simulink model "CoETS_TrqCalc"  (R2016b)
settings: configuration reference "CodeGenConfigSet" (kept outside this file)
values from neighbouring files (symbols this model uses):
  CoETS_trqMaxOfsBrkDes_C = Calibration.Parameter    [init_CoETS_TrqCalc.m]    (also in init_CoETS_TrqCalc_SIL.m = Simulink.Parameter)
  CoETS_trqMinOfsBrkDes_C = Calibration.Parameter    [init_CoETS_TrqCalc.m]    (also in init_CoETS_TrqCalc_SIL.m = Simulink.Parameter)
  DCSOVRDSENGPRT_SY = fi(0,State_int32)    [init_CoETS_TrqCalc.m]    (also in init_CoETS_TrqCalc_SIL.m)
  ENGPRT_OVRDS_DCS = fi(1,State_int32)    [init_CoETS_TrqCalc.m]    (also in init_CoETS_TrqCalc_SIL.m)
  PTPRTOVRDSSPDGOV_SY = fi(0,State_int32)    [init_CoETS_TrqCalc.m]    (also in init_CoETS_TrqCalc_SIL.m)
  SPDGOV_OVRDS_PTPRT = fi(0,State_int32)    [init_CoETS_TrqCalc.m]    (also in init_CoETS_TrqCalc_SIL.m)
libraries: simulink x7
settings Model: Creator=Wollf  LastModifiedBy=xuxingpei
settings ConfigSetRef: SourceLocation=Base Workspace

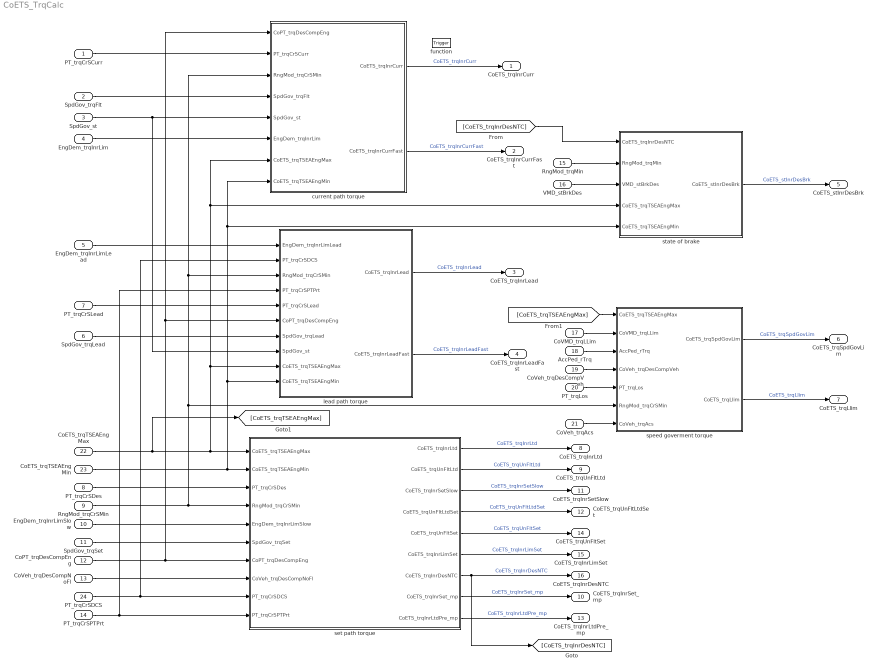
== system CoETS_TrqCalc ==
  PT_trqCrSCurr : Inport  Tag=Nm  Description=application parameter for lead torque order to engine for rail pressure control（crankshaft torque）  OutMin=-3000  OutMax=3000  OutDataTypeStr=Trq_Nm
  SpdGov_trqFlt : Inport  Tag=Nm  Description=filtered setpoint torque of SpdGov  Port=2  OutMin=-3267  OutMax=3267  OutDataTypeStr=Trq_Nm
  SpdGov_st : Inport  Description=status speed control SpdGov  Port=3  OutMin=0  OutMax=65535  OutDataTypeStr=State_uint16
  EngDem_trqInrLim : Inport  Tag=Nm  Description=Resulting limiting torque (inner engine torque)  Port=4  OutMin=-3276.8  OutMax=3276.7  OutDataTypeStr=Trq_Nm
  EngDem_trqInrLimLead : Inport  Tag=Nm  Description=inner engine limted lead torque  Port=5  OutMin=-3276.8  OutMax=3276.7  OutDataTypeStr=Trq_Nm
  SpdGov_trqLead : Inport  Tag=Nm  Description=lead torque of SpdGov on the air path  Port=6  OutMin=-3267  OutMax=3267  OutDataTypeStr=Trq_Nm
  PT_trqCrSLead : Inport  Tag=Nm  Description=application parameter for lead torque order to engine（crankshaft torque）  Port=7  OutMin=-3000  OutMax=3000  OutDataTypeStr=Trq_Nm
  PT_trqCrSDes : Inport  Tag=Nm  Description=Application parameter for requested propulsion torque to engine(crankshaft torque)  Port=8  OutMin=-3000  OutMax=3000  OutDataTypeStr=Trq_Nm
  RngMod_trqCrSMin : Inport  Tag=Nm  Description=minimal crankshaft torque  Port=9  OutMin=-3276.8  OutMax=3276.7  OutDataTypeStr=Trq_Nm
  EngDem_trqInrLimSlow : Inport  Tag=Nm  Description=inner engine limted torque for Slow Path  Port=10  OutMin=-3276.8  OutMax=3276.7  OutDataTypeStr=Trq_Nm
  SpdGov_trqSet : Inport  Tag=Nm  Description=Set point torque of SpdGov on the fuel path  Port=11  OutMin=-3000  OutMax=3000  OutDataTypeStr=Trq_Nm
  CoPT_trqDesCompEng : Inport  Tag=Nm  Description=Application parameter for engine torque desired for compensation  Port=12  OutMin=-3276  OutMax=3276  OutDataTypeStr=Trq_Nm
  CoVeh_trqDesCompNoFl : Inport  Tag=Nm  Description=compensation torque with the shares,which not slur by the drive behaviour filter  Port=13  OutMin=-3000  OutMax=3000  OutDataTypeStr=Trq_Nm
  PT_trqCrSPTPrt : Inport  Tag=Nm  Description=Application parameter for powertrain protection train protection torque(crankshaft torque)  Port=14  OutMin=-3000  OutMax=3000  OutDataTypeStr=Trq_Nm
  RngMod_trqMin : Inport  Tag=Nm  Description=Drag torque (minimum torque)  Port=15  OutMin=-3276.8  OutMax=3276.7  OutDataTypeStr=Trq_Nm
  VMD_stBrkDes : Inport  Description=Application parameter for torque status information  Port=16  OutMin=0  OutMax=65535  OutDataTypeStr=State_uint16
  CoVMD_trqLLim : Inport  Tag=Nm  Description=propulsion torque of longitudinal limter  Port=17  OutMin=-3000  OutMax=3000  OutDataTypeStr=Trq_Nm
  AccPed_rTrq : Inport  Description=Total drive train ratio of engine - wheel  Port=18  OutMin=-327  OutMax=327  OutDataTypeStr=TransRatio
  CoVeh_trqDesCompVeh : Inport  Tag=Nm  Description=Signal for compensation correction of wheel torque level (signal 1)  Port=19  OutMin=-3000  OutMax=3000  OutDataTypeStr=Trq_Nm
  PT_trqLos : Inport  Tag=Nm  Description=Parameter for loss torque of the drive train  Port=20  OutMin=-3000  OutMax=3000  OutDataTypeStr=Trq_Nm
  CoVeh_trqAcs : Inport  Tag=Nm  Description=message for demand of accessories  Port=21  OutMin=-3276.8  OutMax=3276.7  OutDataTypeStr=Trq_Nm
  CoETS_trqTSEAEngMax : Inport  Tag=Nm  Description=torque request to engine intervention decrement(Max)  Port=22  OutMin=-3276  OutMax=3276  OutDataTypeStr=Trq_Nm
  CoETS_trqTSEAEngMin : Inport  Tag=Nm  Description=torque request to engine intervention increment(Min)  Port=23  OutMin=-3276  OutMax=3276  OutDataTypeStr=Trq_Nm
  PT_trqCrSDCS : Inport  Tag=Nm  Description=crankshaft torque for request decrcment  Port=24  OutMin=-3000  OutMax=3000  OutDataTypeStr=Trq_Nm
  function : TriggerPort  TriggerType=function-call  VariantControl=Variant
  current path torque : Subsystem
  lead path torque : Subsystem
  set path torque : Subsystem
  speed goverment torque : Subsystem
  state of brake : Subsystem
  CoETS_trqInrCurr : Outport  Tag=Nm  Description=Inner torque current value  OutMin=-3276  OutMax=3276  OutDataTypeStr=Trq_Nm
  CoETS_trqInrCurrFast : Outport  Tag=Nm  Description=Inner desired torque (fast path) calculated from CoPT_trqCurrEng [Nm]  Port=2  OutMin=-3276  OutMax=3276  OutDataTypeStr=Trq_Nm
  CoETS_trqInrLead : Outport  Tag=Nm  Description=desired lead (inner) torque (without Filter with reserve)  Port=3  OutMin=-3276  OutMax=3276  OutDataTypeStr=Trq_Nm
  CoETS_trqInrLeadFast : Outport  Tag=Nm  Description=Inner torque desired value (fast signal path) generated out of CoPT_trqLeadEng  Port=4  OutMin=-3276  OutMax=3276  OutDataTypeStr=Trq_Nm
  CoETS_stInrDesBrk : Outport  Description=Negative torque status for inner torque  Port=5  OutMin=0  OutMax=4294967295  OutDataTypeStr=State_uint32
  CoETS_trqSpdGovLim : Outport  Tag=Nm  Description=Inner engine limitation torque for EISGov  Port=6  OutMin=-3276.8  OutMax=3276.7  OutDataTypeStr=Trq_Nm
  CoETS_trqLlim : Outport  Tag=Nm  Description=Longitudinal limitation for inner engine torque  Port=7  OutMin=-3276  OutMax=3276  OutDataTypeStr=Trq_Nm
  CoETS_trqInrLtd : Outport  Tag=Nm  Description=inner torque set value after limitation, before AS  Port=8  OutMin=-3000  OutMax=3000  OutDataTypeStr=Trq_Nm
  CoETS_trqUnFltLtd : Outport  Tag=Nm  Description=Limited idle speed governor torque  Port=9  OutMin=-3276  OutMax=3276  OutDataTypeStr=Trq_Nm
  CoETS_trqInrSet_mp : Outport  Tag=Nm  Description=Intermediate inner torque for the set path without filteration  Port=10  OutMin=-3276  OutMax=3276  OutDataTypeStr=Trq_Nm
  CoETS_trqInrSetSlow : Outport  Tag=Nm  Description=Filtered inner torque ( positive torque) desired value (standard signal path) generated out of CoPT_trqDesEng  Port=11  OutMin=-3276  OutMax=3276  OutDataTypeStr=Trq_Nm
  CoETS_trqUnFltLtdSet : Outport  Tag=Nm  Description=Compensation torque of the accessories  Port=12  OutMin=-3276  OutMax=3276  OutDataTypeStr=Trq_Nm
  CoETS_trqInrLtdPre_mp : Outport  Tag=Nm  Description=inner set torque after limitation, before active surge damper  Port=13  OutMin=-3276  OutMax=3276  OutDataTypeStr=Trq_Nm
  CoETS_trqUnFltSet : Outport  Tag=Nm  Description="Compensation torque of \"loss torque compensation\" to bypass filter influences on the set path which is partly compensated"  Port=14  OutMin=-3276  OutMax=3276  OutDataTypeStr=Trq_Nm
  CoETS_trqInrLimSet : Outport  Tag=Nm  Description=Limitation torque without the part of the speed governor  Port=15  OutMin=-3000  OutMax=3000  OutDataTypeStr=Trq_Nm
  CoETS_trqInrDesNTC : Outport  Tag=Nm  Description=Additional desired engine friction Nm  Port=16  OutMin=-3276  OutMax=3276  OutDataTypeStr=Trq_Nm
  wires:
  RngMod_trqMin/1 -> state of brake/2(RngMod_trqMin)
  SpdGov_st/1 -> lead path torque/8(SpdGov_st), current path torque/5(SpdGov_st)
  SpdGov_trqFlt/1 -> current path torque/4(SpdGov_trqFlt)
  EngDem_trqInrLim/1 -> current path torque/6(EngDem_trqInrLim)
  VMD_stBrkDes/1 -> state of brake/3(VMD_stBrkDes)
  state of brake/1(CoETS_stInrDesBrk) -> CoETS_stInrDesBrk/1  "CoETS_stInrDesBrk"
  current path torque/1(CoETS_trqInrCurr) -> CoETS_trqInrCurr/1  "CoETS_trqInrCurr"
  AccPed_rTrq/1 -> speed goverment torque/3(AccPed_rTrq)
  CoVeh_trqAcs/1 -> speed goverment torque/7(CoVeh_trqAcs)
  CoVMD_trqLLim/1 -> speed goverment torque/2(CoVMD_trqLLim)
  speed goverment torque/1(CoETS_trqSpdGovLim) -> CoETS_trqSpdGovLim/1  "CoETS_trqSpdGovLim"
  CoVeh_trqDesCompVeh/1 -> speed goverment torque/4(CoVeh_trqDesCompVeh)
  PT_trqLos/1 -> speed goverment torque/5(PT_trqLos)
  lead path torque/1(CoETS_trqInrLead) -> CoETS_trqInrLead/1  "CoETS_trqInrLead"
  PT_trqCrSCurr/1 -> current path torque/2(PT_trqCrSCurr)
  EngDem_trqInrLimLead/1 -> lead path torque/1(EngDem_trqInrLimLead)
  RngMod_trqCrSMin/1 -> current path torque/3(RngMod_trqCrSMin), lead path torque/3(RngMod_trqCrSMin), speed goverment torque/6(RngMod_trqCrSMin), set path torque/4(RngMod_trqCrSMin)
  CoPT_trqDesCompEng/1 -> current path torque/1(CoPT_trqDesCompEng), lead path torque/6(CoPT_trqDesCompEng), set path torque/7(CoPT_trqDesCompEng)
  PT_trqCrSPTPrt/1 -> lead path torque/4(PT_trqCrSPTPrt), set path torque/10(PT_trqCrSPTPrt)
  CoETS_trqTSEAEngMin/1 -> current path torque/8(CoETS_trqTSEAEngMin), state of brake/5(CoETS_trqTSEAEngMin), lead path torque/10(CoETS_trqTSEAEngMin), set path torque/2(CoETS_trqTSEAEngMin)
  CoETS_trqTSEAEngMax/1 -> [CoETS_trqTSEAEngMax], current path torque/7(CoETS_trqTSEAEngMax), state of brake/4(CoETS_trqTSEAEngMax), lead path torque/9(CoETS_trqTSEAEngMax), set path torque/1(CoETS_trqTSEAEngMax)
  [CoETS_trqInrDesNTC] -> state of brake/1(CoETS_trqInrDesNTC)
  current path torque/2(CoETS_trqInrCurrFast) -> CoETS_trqInrCurrFast/1  "CoETS_trqInrCurrFast"
  lead path torque/2(CoETS_trqInrLeadFast) -> CoETS_trqInrLeadFast/1  "CoETS_trqInrLeadFast"
  speed goverment torque/2(CoETS_trqLlim) -> CoETS_trqLlim/1  "CoETS_trqLlim"
  PT_trqCrSDes/1 -> set path torque/3(PT_trqCrSDes)
  EngDem_trqInrLimSlow/1 -> set path torque/5(EngDem_trqInrLimSlow)
  SpdGov_trqSet/1 -> set path torque/6(SpdGov_trqSet)
  CoVeh_trqDesCompNoFl/1 -> set path torque/8(CoVeh_trqDesCompNoFl)
  set path torque/2(CoETS_trqUnFltLtd) -> CoETS_trqUnFltLtd/1  "CoETS_trqUnFltLtd"
  set path torque/9(CoETS_trqInrLtdPre_mp) -> CoETS_trqInrLtdPre_mp/1  "CoETS_trqInrLtdPre_mp"
  set path torque/6(CoETS_trqInrLimSet) -> CoETS_trqInrLimSet/1  "CoETS_trqInrLimSet"
  set path torque/7(CoETS_trqInrDesNTC) -> CoETS_trqInrDesNTC/1, [CoETS_trqInrDesNTC]  "CoETS_trqInrDesNTC"
  [CoETS_trqTSEAEngMax] -> speed goverment torque/1(CoETS_trqTSEAEngMax)
  set path torque/8(CoETS_trqInrSet_mp) -> CoETS_trqInrSet_mp/1  "CoETS_trqInrSet_mp"
  set path torque/3(CoETS_trqInrSetSlow) -> CoETS_trqInrSetSlow/1  "CoETS_trqInrSetSlow"
  set path torque/1(CoETS_trqInrLtd) -> CoETS_trqInrLtd/1  "CoETS_trqInrLtd"
  PT_trqCrSDCS/1 -> lead path torque/2(PT_trqCrSDCS), set path torque/9(PT_trqCrSDCS)
  set path torque/4(CoETS_trqUnFltLtdSet) -> CoETS_trqUnFltLtdSet/1  "CoETS_trqUnFltLtdSet"
  set path torque/5(CoETS_trqUnFltSet) -> CoETS_trqUnFltSet/1  "CoETS_trqUnFltSet"
  SpdGov_trqLead/1 -> lead path torque/7(SpdGov_trqLead)
  PT_trqCrSLead/1 -> lead path torque/5(PT_trqCrSLead)

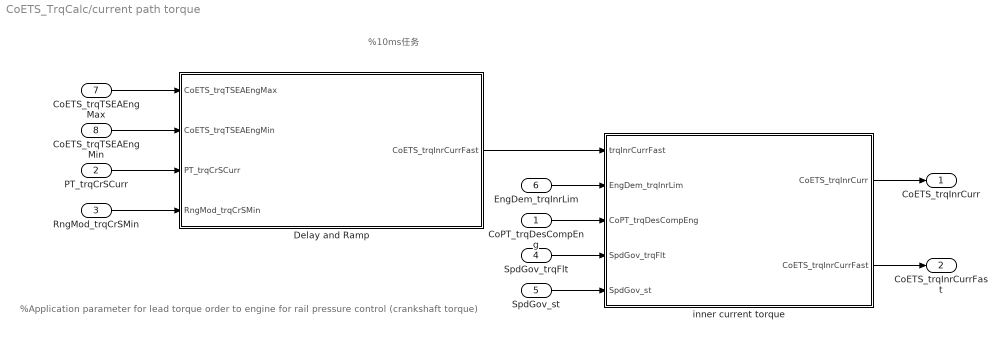
== system CoETS_TrqCalc/current path torque ==
  note: %10ms任务
  note: %Application parameter for lead torque order to engine for rail pressure control (crankshaft torque)
  CoPT_trqDesCompEng : Inport
  PT_trqCrSCurr : Inport  Port=2
  RngMod_trqCrSMin : Inport  Port=3
  SpdGov_trqFlt : Inport  Port=4
  SpdGov_st : Inport  Port=5
  EngDem_trqInrLim : Inport  Port=6
  CoETS_trqTSEAEngMax : Inport  Port=7
  CoETS_trqTSEAEngMin : Inport  Port=8
  Delay and Ramp : Subsystem
  inner current torque : Subsystem
  CoETS_trqInrCurr : Outport
  CoETS_trqInrCurrFast : Outport  Port=2
  wires:
  RngMod_trqCrSMin/1 -> Delay and Ramp/4(RngMod_trqCrSMin)
  PT_trqCrSCurr/1 -> Delay and Ramp/3(PT_trqCrSCurr)
  CoETS_trqTSEAEngMin/1 -> Delay and Ramp/2(CoETS_trqTSEAEngMin)
  CoETS_trqTSEAEngMax/1 -> Delay and Ramp/1(CoETS_trqTSEAEngMax)
  Delay and Ramp/1(CoETS_trqInrCurrFast) -> inner current torque/1(trqInrCurrFast)
  EngDem_trqInrLim/1 -> inner current torque/2(EngDem_trqInrLim)
  CoPT_trqDesCompEng/1 -> inner current torque/3(CoPT_trqDesCompEng)
  SpdGov_trqFlt/1 -> inner current torque/4(SpdGov_trqFlt)
  SpdGov_st/1 -> inner current torque/5(SpdGov_st)
  inner current torque/1(CoETS_trqInrCurr) -> CoETS_trqInrCurr/1
  inner current torque/2(CoETS_trqInrCurrFast) -> CoETS_trqInrCurrFast/1

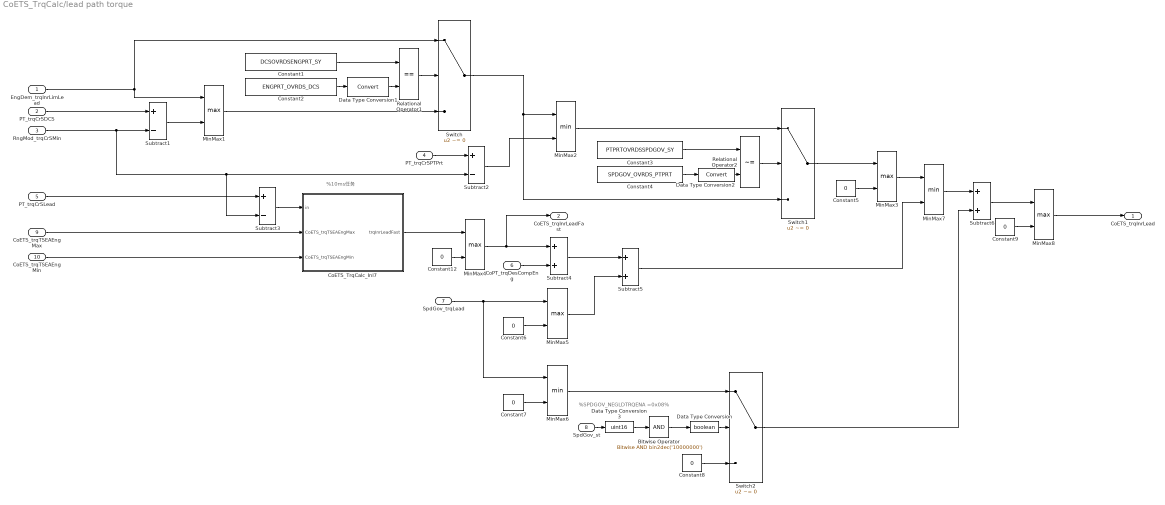
== system CoETS_TrqCalc/lead path torque ==
  note: %10ms任务
  note: %SPDGOV_NEGLDTRQENA =0x08%
  EngDem_trqInrLimLead : Inport
  PT_trqCrSDCS : Inport  Port=2
  RngMod_trqCrSMin : Inport  Port=3
  PT_trqCrSPTPrt : Inport  Port=4
  PT_trqCrSLead : Inport  Port=5
  CoPT_trqDesCompEng : Inport  Port=6
  SpdGov_trqLead : Inport  Port=7
  SpdGov_st : Inport  Port=8
  CoETS_trqTSEAEngMax : Inport  Port=9
  CoETS_trqTSEAEngMin : Inport  Port=10
  Bitwise Operator : simulink/Logic and Bit Operations/Bitwise Operator  logicop=AND  UseBitMask=on  BitMask=bin2dec('10000000')  BitMaskRealWorld=Stored Integer
  CoETS_TrqCalc_Inl7 : Subsystem
  Constant1 : Constant  Value=DCSOVRDSENGPRT_SY  VectorParams1D=off
  Constant{5..9,12} (6 alike) : Constant  Value=0  VectorParams1D=off  OutDataTypeStr=Inherit: Inherit via back propagation
  Constant2 : Constant  Value=ENGPRT_OVRDS_DCS  VectorParams1D=off
  Constant3 : Constant  Value=PTPRTOVRDSSPDGOV_SY  VectorParams1D=off
  Constant4 : Constant  Value=SPDGOV_OVRDS_PTPRT  VectorParams1D=off
  Data Type Conversion : DataTypeConversion  OutDataTypeStr=boolean
  Data Type Conversion1 : DataTypeConversion
  Data Type Conversion2 : DataTypeConversion
  Data Type Conversion3 : DataTypeConversion  OutDataTypeStr=uint16
  MinMax{1,3..5,8} (5 alike) : MinMax  Function=max  Inputs=2  InputSameDT=on
  MinMax2 : MinMax  Inputs=2  InputSameDT=on
  MinMax6 : MinMax  Inputs=2  InputSameDT=on
  MinMax7 : MinMax  Inputs=2  InputSameDT=on
  Relational Operator1 : RelationalOperator  Operator===  OutDataTypeStr=boolean  RndMeth=Simplest  InputSameDT=on
  Relational Operator2 : RelationalOperator  Operator=~=  OutDataTypeStr=boolean  RndMeth=Simplest  InputSameDT=on
  Subtract1 : Sum  Inputs=+-  OutDataTypeStr=Inherit: Inherit via back propagation  SaturateOnIntegerOverflow=on  InputSameDT=on
  Subtract2 : Sum  Inputs=+-  OutDataTypeStr=Inherit: Inherit via back propagation  SaturateOnIntegerOverflow=on  InputSameDT=on
  Subtract3 : Sum  Inputs=+-  OutDataTypeStr=Inherit: Inherit via back propagation  SaturateOnIntegerOverflow=on  InputSameDT=on
  Subtract4 : Sum  OutDataTypeStr=Inherit: Inherit via back propagation  SaturateOnIntegerOverflow=on  InputSameDT=on
  Subtract5 : Sum  OutDataTypeStr=Inherit: Inherit via back propagation  SaturateOnIntegerOverflow=on  InputSameDT=on
  Subtract6 : Sum  OutDataTypeStr=Inherit: Inherit via back propagation  SaturateOnIntegerOverflow=on  InputSameDT=on
  Switch : Switch  Criteria=u2 ~= 0  OutDataTypeStr=Inherit: Inherit via back propagation  SaturateOnIntegerOverflow=on  InputSameDT=on
  Switch1 : Switch  Criteria=u2 ~= 0  OutDataTypeStr=Inherit: Inherit via back propagation  SaturateOnIntegerOverflow=on  InputSameDT=on
  Switch2 : Switch  Criteria=u2 ~= 0  OutDataTypeStr=Inherit: Inherit via back propagation  SaturateOnIntegerOverflow=on  InputSameDT=on
  CoETS_trqInrLead : Outport
  CoETS_trqInrLeadFast : Outport  Port=2
  wires:
  EngDem_trqInrLimLead/1 -> MinMax1/1, Switch/1
  Subtract1/1 -> MinMax1/2
  MinMax1/1 -> Switch/3
  Data Type Conversion2/1 -> Relational Operator2/2
  Data Type Conversion1/1 -> Relational Operator1/2
  CoETS_trqTSEAEngMin/1 -> CoETS_TrqCalc_Inl7/3(CoETS_trqTSEAEngMin)
  CoETS_trqTSEAEngMax/1 -> CoETS_TrqCalc_Inl7/2(CoETS_trqTSEAEngMax)
  MinMax8/1 -> CoETS_trqInrLead/1
  Constant9/1 -> MinMax8/2
  Subtract6/1 -> MinMax8/1
  Switch2/1 -> Subtract6/2
  MinMax7/1 -> Subtract6/1
  Subtract5/1 -> MinMax7/2
  MinMax3/1 -> MinMax7/1
  Constant8/1 -> Switch2/3
  Data Type Conversion/1 -> Switch2/2
  Bitwise Operator/1 -> Data Type Conversion/1
  SpdGov_st/1 -> Data Type Conversion3/1
  MinMax6/1 -> Switch2/1
  MinMax5/1 -> Subtract5/2
  Subtract4/1 -> Subtract5/1
  SpdGov_trqLead/1 -> MinMax5/1, MinMax6/1
  Constant7/1 -> MinMax6/2
  Constant6/1 -> MinMax5/2
  CoPT_trqDesCompEng/1 -> Subtract4/2
  MinMax4/1 -> Subtract4/1, CoETS_trqInrLeadFast/1
  Constant12/1 -> MinMax4/2
  CoETS_TrqCalc_Inl7/1(trqInrLeadFast) -> MinMax4/1
  Subtract3/1 -> CoETS_TrqCalc_Inl7/1(in)
  PT_trqCrSLead/1 -> Subtract3/1
  Constant5/1 -> MinMax3/2
  Switch1/1 -> MinMax3/1
  MinMax2/1 -> Switch1/1
  Subtract2/1 -> MinMax2/2
  PT_trqCrSPTPrt/1 -> Subtract2/1
  Switch/1 -> MinMax2/1, Switch1/3
  RngMod_trqCrSMin/1 -> Subtract1/2, Subtract3/2, Subtract2/2
  PT_trqCrSDCS/1 -> Subtract1/1
  Relational Operator2/1 -> Switch1/2
  Relational Operator1/1 -> Switch/2
  Constant4/1 -> Data Type Conversion2/1
  Constant3/1 -> Relational Operator2/1
  Constant2/1 -> Data Type Conversion1/1
  Constant1/1 -> Relational Operator1/1
  Data Type Conversion3/1 -> Bitwise Operator/1

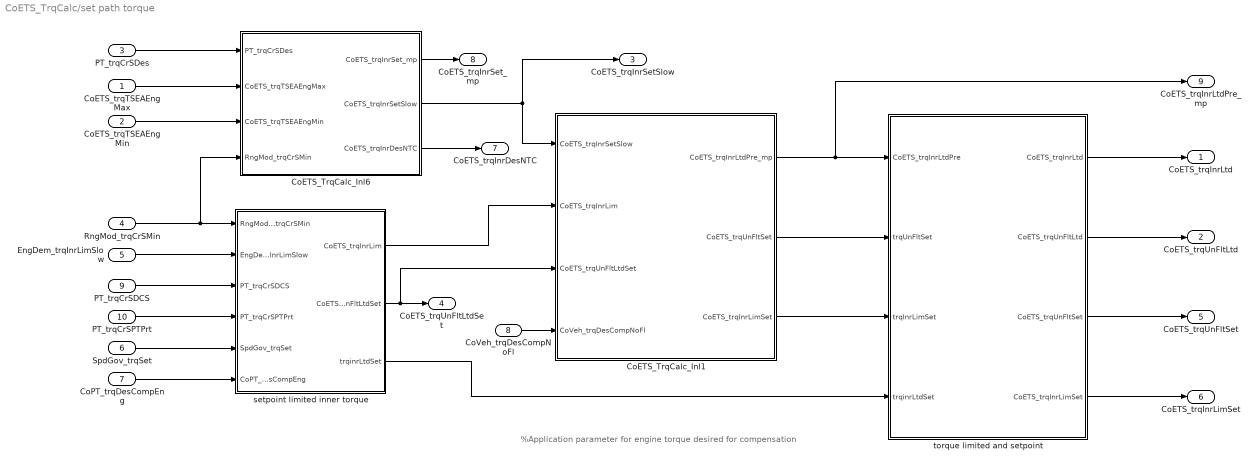
== system CoETS_TrqCalc/set path torque ==
  note: %Application parameter for engine torque desired for compensation
  CoETS_trqTSEAEngMax : Inport
  CoETS_trqTSEAEngMin : Inport  Port=2
  PT_trqCrSDes : Inport  Port=3
  RngMod_trqCrSMin : Inport  Port=4
  EngDem_trqInrLimSlow : Inport  Port=5
  SpdGov_trqSet : Inport  Port=6
  CoPT_trqDesCompEng : Inport  Port=7
  CoVeh_trqDesCompNoFl : Inport  Port=8
  PT_trqCrSDCS : Inport  Port=9
  PT_trqCrSPTPrt : Inport  Port=10
  CoETS_TrqCalc_Inl1 : Subsystem
  CoETS_TrqCalc_Inl6 : Subsystem
  setpoint limited inner torque : Subsystem
  torque limited and setpoint : Subsystem
  CoETS_trqInrLtd : Outport
  CoETS_trqUnFltLtd : Outport  Port=2
  CoETS_trqInrSetSlow : Outport  Port=3
  CoETS_trqUnFltLtdSet : Outport  Port=4
  CoETS_trqUnFltSet : Outport  Port=5
  CoETS_trqInrLimSet : Outport  Port=6
  CoETS_trqInrDesNTC : Outport  Port=7
  CoETS_trqInrSet_mp : Outport  Port=8
  CoETS_trqInrLtdPre_mp : Outport  Port=9
  wires:
  RngMod_trqCrSMin/1 -> CoETS_TrqCalc_Inl6/4(RngMod_trqCrSMin), setpoint limited inner torque/1(RngMod_trqCrSMin)
  PT_trqCrSDes/1 -> CoETS_TrqCalc_Inl6/1(PT_trqCrSDes)
  CoETS_trqTSEAEngMax/1 -> CoETS_TrqCalc_Inl6/2(CoETS_trqTSEAEngMax)
  CoETS_trqTSEAEngMin/1 -> CoETS_TrqCalc_Inl6/3(CoETS_trqTSEAEngMin)
  CoVeh_trqDesCompNoFl/1 -> CoETS_TrqCalc_Inl1/4(CoVeh_trqDesCompNoFl)
  setpoint limited inner torque/2(CoETS_trqUnFltLtdSet) -> CoETS_trqUnFltLtdSet/1, CoETS_TrqCalc_Inl1/3(CoETS_trqUnFltLtdSet)
  EngDem_trqInrLimSlow/1 -> setpoint limited inner torque/2(EngDem_trqInrLimSlow)
  PT_trqCrSDCS/1 -> setpoint limited inner torque/3(PT_trqCrSDCS)
  PT_trqCrSPTPrt/1 -> setpoint limited inner torque/4(PT_trqCrSPTPrt)
  SpdGov_trqSet/1 -> setpoint limited inner torque/5(SpdGov_trqSet)
  CoPT_trqDesCompEng/1 -> setpoint limited inner torque/6(CoPT_trqDesCompEng)
  setpoint limited inner torque/1(CoETS_trqInrLim) -> CoETS_TrqCalc_Inl1/2(CoETS_trqInrLim)
  CoETS_TrqCalc_Inl6/1(CoETS_trqInrSet_mp) -> CoETS_trqInrSet_mp/1
  CoETS_TrqCalc_Inl6/2(CoETS_trqInrSetSlow) -> CoETS_trqInrSetSlow/1, CoETS_TrqCalc_Inl1/1(CoETS_trqInrSetSlow)
  CoETS_TrqCalc_Inl6/3(CoETS_trqInrDesNTC) -> CoETS_trqInrDesNTC/1
  CoETS_TrqCalc_Inl1/1(CoETS_trqInrLtdPre_mp) -> CoETS_trqInrLtdPre_mp/1, torque limited and setpoint/1(CoETS_trqInrLtdPre)
  CoETS_TrqCalc_Inl1/2(CoETS_trqUnFltSet) -> torque limited and setpoint/2(trqUnFltSet)
  CoETS_TrqCalc_Inl1/3(CoETS_trqInrLimSet) -> torque limited and setpoint/3(trqInrLimSet)
  setpoint limited inner torque/3(trqinrLtdSet) -> torque limited and setpoint/4(trqinrLtdSet)
  torque limited and setpoint/1(CoETS_trqInrLtd) -> CoETS_trqInrLtd/1
  torque limited and setpoint/2(CoETS_trqUnFltLtd) -> CoETS_trqUnFltLtd/1
  torque limited and setpoint/3(CoETS_trqUnFltSet) -> CoETS_trqUnFltSet/1
  torque limited and setpoint/4(CoETS_trqInrLimSet) -> CoETS_trqInrLimSet/1

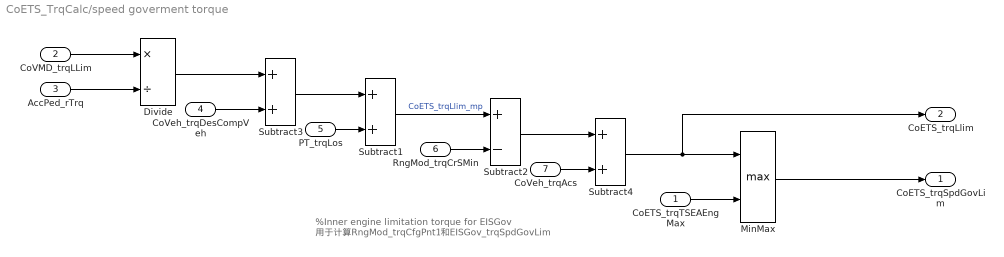
== system CoETS_TrqCalc/speed goverment torque ==
  note: %Inner engine limitation torque for EISGov
      | 用于计算RngMod_trqCfgPnt1和EISGov_trqSpdGovLim
  CoETS_trqTSEAEngMax : Inport
  CoVMD_trqLLim : Inport  Port=2
  AccPed_rTrq : Inport  Port=3
  CoVeh_trqDesCompVeh : Inport  Port=4
  PT_trqLos : Inport  Port=5
  RngMod_trqCrSMin : Inport  Port=6
  CoVeh_trqAcs : Inport  Port=7
  Divide : Product  Inputs=*/  OutDataTypeStr=Inherit: Inherit via back propagation  SaturateOnIntegerOverflow=on
  MinMax : MinMax  Function=max  Inputs=2  InputSameDT=on
  Subtract1 : Sum  OutDataTypeStr=Inherit: Inherit via back propagation  SaturateOnIntegerOverflow=on  InputSameDT=on
  Subtract2 : Sum  Inputs=+-  OutDataTypeStr=Inherit: Inherit via back propagation  SaturateOnIntegerOverflow=on  InputSameDT=on
  Subtract3 : Sum  OutDataTypeStr=Inherit: Inherit via back propagation  SaturateOnIntegerOverflow=on  InputSameDT=on
  Subtract4 : Sum  OutDataTypeStr=Inherit: Inherit via back propagation  SaturateOnIntegerOverflow=on  InputSameDT=on
  CoETS_trqSpdGovLim : Outport
  CoETS_trqLlim : Outport  Port=2
  wires:
  MinMax/1 -> CoETS_trqSpdGovLim/1
  CoETS_trqTSEAEngMax/1 -> MinMax/2
  Subtract4/1 -> MinMax/1, CoETS_trqLlim/1
  CoVeh_trqAcs/1 -> Subtract4/2
  Subtract2/1 -> Subtract4/1
  RngMod_trqCrSMin/1 -> Subtract2/2
  Subtract1/1 -> Subtract2/1  "CoETS_trqLlim_mp"
  PT_trqLos/1 -> Subtract1/2
  Subtract3/1 -> Subtract1/1
  CoVeh_trqDesCompVeh/1 -> Subtract3/2
  Divide/1 -> Subtract3/1
  AccPed_rTrq/1 -> Divide/2
  CoVMD_trqLLim/1 -> Divide/1

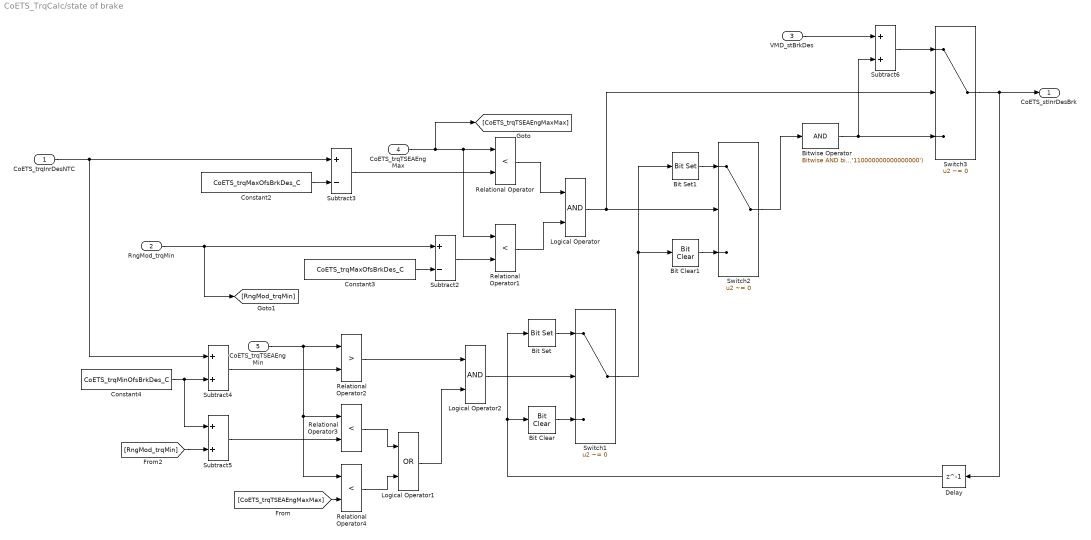
== system CoETS_TrqCalc/state of brake ==
  CoETS_trqInrDesNTC : Inport
  RngMod_trqMin : Inport  Port=2
  VMD_stBrkDes : Inport  Port=3
  CoETS_trqTSEAEngMax : Inport  Port=4
  CoETS_trqTSEAEngMin : Inport  Port=5
  Bit Clear : simulink/Logic and Bit Operations/Bit Clear  iBit=17
  Bit Clear1 : simulink/Logic and Bit Operations/Bit Clear  iBit=16
  Bit Set : simulink/Logic and Bit Operations/Bit Set  iBit=17
  Bit Set1 : simulink/Logic and Bit Operations/Bit Set  iBit=16
  Bitwise Operator : simulink/Logic and Bit Operations/Bitwise Operator  logicop=AND  UseBitMask=on  BitMask=bin2dec('110000000000000000')  BitMaskRealWorld=Stored Integer
  Constant2 : Constant  Value=CoETS_trqMaxOfsBrkDes_C  VectorParams1D=off
  Constant3 : Constant  Value=CoETS_trqMaxOfsBrkDes_C  VectorParams1D=off
  Constant4 : Constant  Value=CoETS_trqMinOfsBrkDes_C  VectorParams1D=off
  Delay : Delay  DelayLength=1  InitialCondition=0
  Logical Operator : Logic  AllPortsSameDT=off  OutDataTypeStr=boolean
  Logical Operator1 : Logic  Operator=OR  AllPortsSameDT=off  OutDataTypeStr=boolean
  Logical Operator2 : Logic  AllPortsSameDT=off  OutDataTypeStr=boolean
  Relational Operator{,1,3..4} (4 alike) : RelationalOperator  Operator=<  OutDataTypeStr=boolean  RndMeth=Simplest  InputSameDT=on
  Relational Operator2 : RelationalOperator  Operator=>  OutDataTypeStr=boolean  RndMeth=Simplest  InputSameDT=on
  Subtract2 : Sum  Inputs=+-  OutDataTypeStr=Inherit: Inherit via back propagation  SaturateOnIntegerOverflow=on  InputSameDT=on
  Subtract3 : Sum  Inputs=+-  OutDataTypeStr=Inherit: Inherit via back propagation  SaturateOnIntegerOverflow=on  InputSameDT=on
  Subtract4 : Sum  OutDataTypeStr=Inherit: Inherit via back propagation  SaturateOnIntegerOverflow=on  InputSameDT=on
  Subtract5 : Sum  OutDataTypeStr=Inherit: Inherit via back propagation  SaturateOnIntegerOverflow=on  InputSameDT=on
  Subtract6 : Sum  OutDataTypeStr=Inherit: Inherit via back propagation  SaturateOnIntegerOverflow=on
  Switch1 : Switch  Criteria=u2 ~= 0  OutDataTypeStr=Inherit: Inherit via back propagation  SaturateOnIntegerOverflow=on  InputSameDT=on
  Switch2 : Switch  Criteria=u2 ~= 0  OutDataTypeStr=Inherit: Inherit via back propagation  SaturateOnIntegerOverflow=on  InputSameDT=on
  Switch3 : Switch  Criteria=u2 ~= 0  OutDataTypeStr=Inherit: Inherit via back propagation  SaturateOnIntegerOverflow=on  InputSameDT=on
  CoETS_stInrDesBrk : Outport
  wires:
  Delay/1 -> Bit Clear/1, Bit Set/1
  VMD_stBrkDes/1 -> Subtract6/1
  Switch2/1 -> Bitwise Operator/1
  Bitwise Operator/1 -> Switch3/3, Subtract6/2
  Subtract6/1 -> Switch3/1
  Switch1/1 -> Bit Clear1/1, Bit Set1/1
  Bit Clear1/1 -> Switch2/3
  Bit Set1/1 -> Switch2/1
  Logical Operator/1 -> Switch2/2, Switch3/2
  Bit Clear/1 -> Switch1/3
  Switch3/1 -> CoETS_stInrDesBrk/1, Delay/1
  Bit Set/1 -> Switch1/1
  Logical Operator2/1 -> Switch1/2
  Logical Operator1/1 -> Logical Operator2/2
  Relational Operator2/1 -> Logical Operator2/1
  Relational Operator3/1 -> Logical Operator1/1
  Relational Operator4/1 -> Logical Operator1/2
  Subtract5/1 -> Relational Operator3/2
  CoETS_trqTSEAEngMin/1 -> Relational Operator2/1, Relational Operator3/1, Relational Operator4/1
  Subtract4/1 -> Relational Operator2/2
  Constant4/1 -> Subtract4/2, Subtract5/1
  CoETS_trqInrDesNTC/1 -> Subtract4/1, Subtract3/1
  Relational Operator1/1 -> Logical Operator/2
  Subtract2/1 -> Relational Operator1/2
  Constant3/1 -> Subtract2/2
  RngMod_trqMin/1 -> [RngMod_trqMin], Subtract2/1
  Relational Operator/1 -> Logical Operator/1
  CoETS_trqTSEAEngMax/1 -> [CoETS_trqTSEAEngMaxMax], Relational Operator/1, Relational Operator1/1
  Subtract3/1 -> Relational Operator/2
  Constant2/1 -> Subtract3/2
  [CoETS_trqTSEAEngMaxMax] -> Relational Operator4/2
  [RngMod_trqMin] -> Subtract5/2

== system CoETS_TrqCalc/current path torque/Delay and Ramp ==
  CoETS_trqTSEAEngMax : Inport
  CoETS_trqTSEAEngMin : Inport  Port=2
  PT_trqCrSCurr : Inport  Port=3
  RngMod_trqCrSMin : Inport  Port=4
  MinMax2 : MinMax  Inputs=2  InputSameDT=on
  MinMax3 : MinMax  Function=max  Inputs=2  InputSameDT=on
  Subtract3 : Sum  Inputs=+-  OutDataTypeStr=Inherit: Inherit via back propagation  SaturateOnIntegerOverflow=on  InputSameDT=on
  CoETS_trqInrCurrFast : Outport
  wires:
  MinMax3/1 -> CoETS_trqInrCurrFast/1
  CoETS_trqTSEAEngMin/1 -> MinMax3/2
  MinMax2/1 -> MinMax3/1
  CoETS_trqTSEAEngMax/1 -> MinMax2/1
  Subtract3/1 -> MinMax2/2
  RngMod_trqCrSMin/1 -> Subtract3/2
  PT_trqCrSCurr/1 -> Subtract3/1

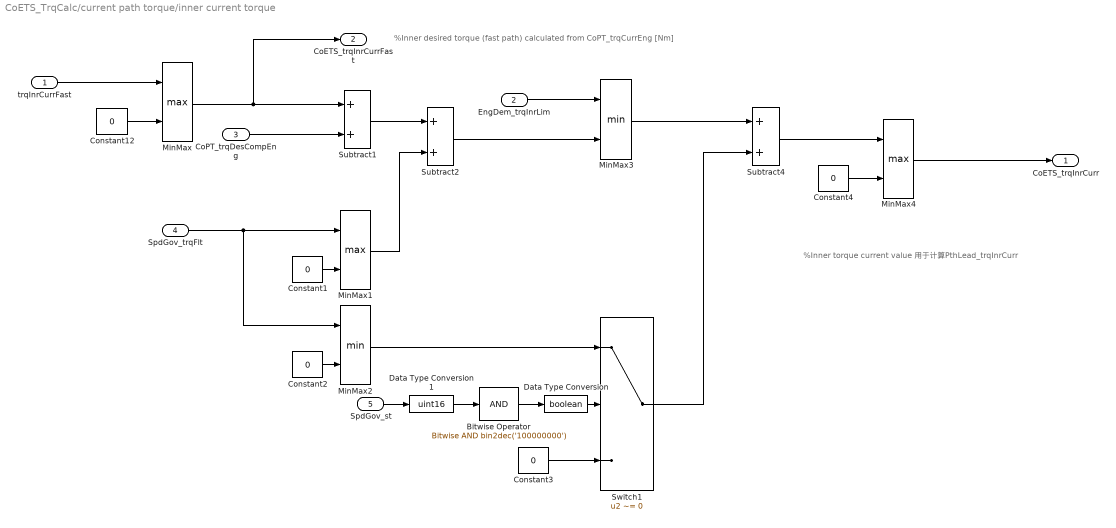
== system CoETS_TrqCalc/current path torque/inner current torque ==
  note: %Inner torque current value 用于计算PthLead_trqInrCurr
  note: %Inner desired torque (fast path) calculated from CoPT_trqCurrEng [Nm]
  trqInrCurrFast : Inport
  EngDem_trqInrLim : Inport  Port=2
  CoPT_trqDesCompEng : Inport  Port=3
  SpdGov_trqFlt : Inport  Port=4
  SpdGov_st : Inport  Port=5
  Bitwise Operator : simulink/Logic and Bit Operations/Bitwise Operator  logicop=AND  UseBitMask=on  BitMask=bin2dec('100000000')  BitMaskRealWorld=Stored Integer
  Constant{1..4,12} (5 alike) : Constant  Value=0  VectorParams1D=off  OutDataTypeStr=Inherit: Inherit via back propagation
  Data Type Conversion : DataTypeConversion  OutDataTypeStr=boolean
  Data Type Conversion1 : DataTypeConversion  OutDataTypeStr=uint16
  MinMax : MinMax  Function=max  Inputs=2  InputSameDT=on
  MinMax1 : MinMax  Function=max  Inputs=2  InputSameDT=on
  MinMax2 : MinMax  Inputs=2  InputSameDT=on
  MinMax3 : MinMax  Inputs=2  OutDataTypeStr=Trq_Nm  InputSameDT=on
  MinMax4 : MinMax  Function=max  Inputs=2  InputSameDT=on
  Subtract1 : Sum  OutDataTypeStr=Inherit: Inherit via back propagation  SaturateOnIntegerOverflow=on  InputSameDT=on
  Subtract2 : Sum  OutDataTypeStr=Inherit: Inherit via back propagation  SaturateOnIntegerOverflow=on  InputSameDT=on
  Subtract4 : Sum  OutDataTypeStr=Inherit: Inherit via back propagation  SaturateOnIntegerOverflow=on  InputSameDT=on
  Switch1 : Switch  Criteria=u2 ~= 0  SaturateOnIntegerOverflow=on  InputSameDT=on
  CoETS_trqInrCurr : Outport
  CoETS_trqInrCurrFast : Outport  Port=2
  wires:
  MinMax3/1 -> Subtract4/1
  EngDem_trqInrLim/1 -> MinMax3/1
  Constant3/1 -> Switch1/3
  Data Type Conversion/1 -> Switch1/2
  MinMax1/1 -> Subtract2/2
  SpdGov_trqFlt/1 -> MinMax1/1, MinMax2/1
  Bitwise Operator/1 -> Data Type Conversion/1
  Constant1/1 -> MinMax1/2
  Constant4/1 -> MinMax4/2
  Switch1/1 -> Subtract4/2
  Constant2/1 -> MinMax2/2
  MinMax4/1 -> CoETS_trqInrCurr/1
  Subtract4/1 -> MinMax4/1
  Subtract2/1 -> MinMax3/2
  MinMax2/1 -> Switch1/1
  SpdGov_st/1 -> Data Type Conversion1/1
  trqInrCurrFast/1 -> MinMax/1
  MinMax/1 -> CoETS_trqInrCurrFast/1, Subtract1/1
  Constant12/1 -> MinMax/2
  Subtract1/1 -> Subtract2/1
  CoPT_trqDesCompEng/1 -> Subtract1/2
  Data Type Conversion1/1 -> Bitwise Operator/1

== system CoETS_TrqCalc/lead path torque/CoETS_TrqCalc_Inl7 ==
  in : Inport
  CoETS_trqTSEAEngMax : Inport  Port=2
  CoETS_trqTSEAEngMin : Inport  Port=3
  MinMax2 : MinMax  Inputs=2  InputSameDT=on
  MinMax3 : MinMax  Function=max  Inputs=2  InputSameDT=on
  trqInrLeadFast : Outport
  wires:
  MinMax3/1 -> trqInrLeadFast/1
  CoETS_trqTSEAEngMin/1 -> MinMax3/2
  MinMax2/1 -> MinMax3/1
  CoETS_trqTSEAEngMax/1 -> MinMax2/1
  in/1 -> MinMax2/2

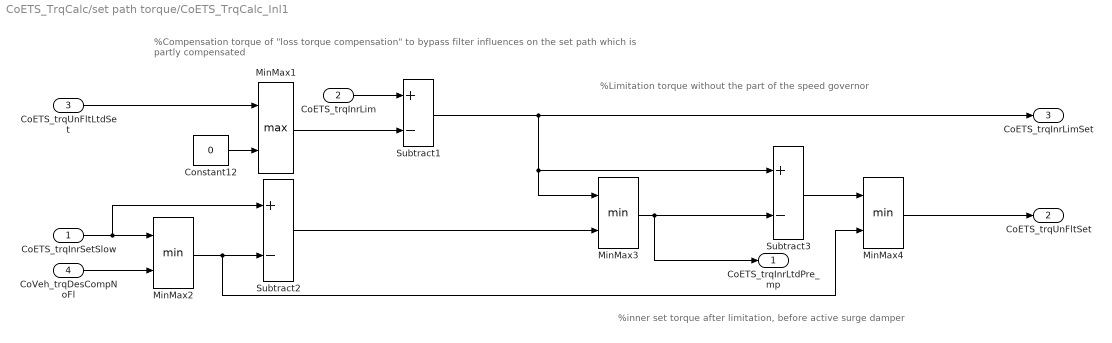
== system CoETS_TrqCalc/set path torque/CoETS_TrqCalc_Inl1 ==
  note: %Limitation torque without the part of the speed governor
  note: %inner set torque after limitation, before active surge damper
  note: %Compensation torque of "loss torque compensation" to bypass filter influences on the set path which is partly compensated
  CoETS_trqInrSetSlow : Inport
  CoETS_trqInrLim : Inport  Port=2
  CoETS_trqUnFltLtdSet : Inport  Port=3
  CoVeh_trqDesCompNoFl : Inport  Port=4
  Constant12 : Constant  Value=0  VectorParams1D=off  OutDataTypeStr=Inherit: Inherit via back propagation
  MinMax1 : MinMax  Function=max  Inputs=2  InputSameDT=on
  MinMax2 : MinMax  Inputs=2  InputSameDT=on
  MinMax3 : MinMax  Inputs=2  InputSameDT=on
  MinMax4 : MinMax  Inputs=2  InputSameDT=on
  Subtract1 : Sum  Inputs=+-  OutDataTypeStr=Inherit: Inherit via back propagation  SaturateOnIntegerOverflow=on  InputSameDT=on
  Subtract2 : Sum  Inputs=+-  OutDataTypeStr=Inherit: Inherit via back propagation  SaturateOnIntegerOverflow=on  InputSameDT=on
  Subtract3 : Sum  Inputs=+-  OutDataTypeStr=Inherit: Inherit via back propagation  SaturateOnIntegerOverflow=on  InputSameDT=on
  CoETS_trqInrLtdPre_mp : Outport
  CoETS_trqUnFltSet : Outport  Port=2
  CoETS_trqInrLimSet : Outport  Port=3
  wires:
  MinMax4/1 -> CoETS_trqUnFltSet/1
  Subtract3/1 -> MinMax4/1
  MinMax3/1 -> CoETS_trqInrLtdPre_mp/1, Subtract3/2
  Subtract1/1 -> CoETS_trqInrLimSet/1, Subtract3/1, MinMax3/1
  Subtract2/1 -> MinMax3/2
  MinMax2/1 -> Subtract2/2, MinMax4/2
  CoVeh_trqDesCompNoFl/1 -> MinMax2/2
  CoETS_trqInrSetSlow/1 -> MinMax2/1, Subtract2/1
  MinMax1/1 -> Subtract1/2
  CoETS_trqUnFltLtdSet/1 -> MinMax1/1
  Constant12/1 -> MinMax1/2
  CoETS_trqInrLim/1 -> Subtract1/1

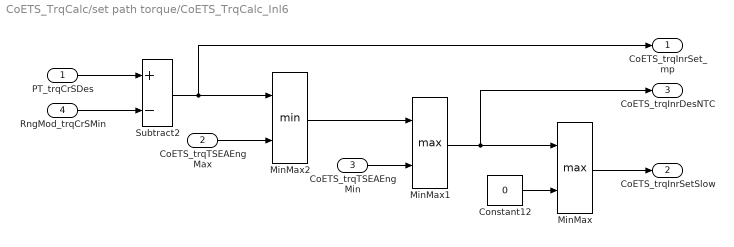
== system CoETS_TrqCalc/set path torque/CoETS_TrqCalc_Inl6 ==
  PT_trqCrSDes : Inport
  CoETS_trqTSEAEngMax : Inport  Port=2
  CoETS_trqTSEAEngMin : Inport  Port=3
  RngMod_trqCrSMin : Inport  Port=4
  Constant12 : Constant  Value=0  VectorParams1D=off  OutDataTypeStr=Inherit: Inherit via back propagation
  MinMax : MinMax  Function=max  Inputs=2  InputSameDT=on
  MinMax1 : MinMax  Function=max  Inputs=2  InputSameDT=on
  MinMax2 : MinMax  Inputs=2  InputSameDT=on
  Subtract2 : Sum  Inputs=+-  OutDataTypeStr=Inherit: Inherit via back propagation  SaturateOnIntegerOverflow=on  InputSameDT=on
  CoETS_trqInrSet_mp : Outport
  CoETS_trqInrSetSlow : Outport  Port=2
  CoETS_trqInrDesNTC : Outport  Port=3
  wires:
  CoETS_trqTSEAEngMin/1 -> MinMax1/2
  RngMod_trqCrSMin/1 -> Subtract2/2
  PT_trqCrSDes/1 -> Subtract2/1
  Subtract2/1 -> MinMax2/1, CoETS_trqInrSet_mp/1
  MinMax/1 -> CoETS_trqInrSetSlow/1
  Constant12/1 -> MinMax/2
  MinMax1/1 -> MinMax/1, CoETS_trqInrDesNTC/1
  CoETS_trqTSEAEngMax/1 -> MinMax2/2
  MinMax2/1 -> MinMax1/1

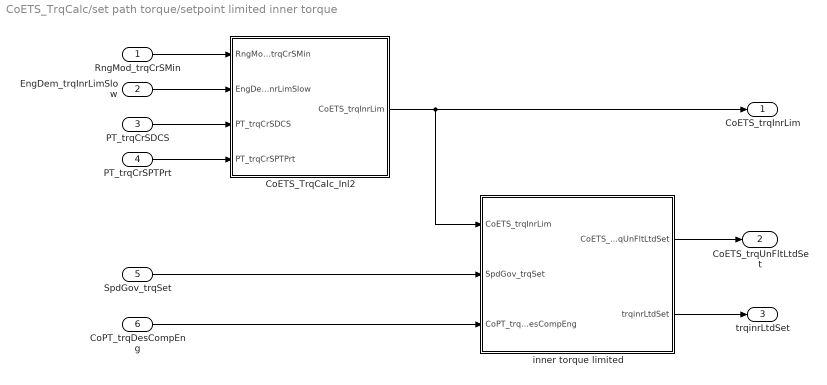
== system CoETS_TrqCalc/set path torque/setpoint limited inner torque ==
  RngMod_trqCrSMin : Inport
  EngDem_trqInrLimSlow : Inport  Port=2
  PT_trqCrSDCS : Inport  Port=3
  PT_trqCrSPTPrt : Inport  Port=4
  SpdGov_trqSet : Inport  Port=5
  CoPT_trqDesCompEng : Inport  Port=6
  CoETS_TrqCalc_Inl2 : Subsystem
  inner torque limited : Subsystem
  CoETS_trqInrLim : Outport
  CoETS_trqUnFltLtdSet : Outport  Port=2
  trqinrLtdSet : Outport  Port=3
  wires:
  EngDem_trqInrLimSlow/1 -> CoETS_TrqCalc_Inl2/2(EngDem_trqInrLimSlow)
  PT_trqCrSPTPrt/1 -> CoETS_TrqCalc_Inl2/4(PT_trqCrSPTPrt)
  PT_trqCrSDCS/1 -> CoETS_TrqCalc_Inl2/3(PT_trqCrSDCS)
  RngMod_trqCrSMin/1 -> CoETS_TrqCalc_Inl2/1(RngMod_trqCrSMin)
  SpdGov_trqSet/1 -> inner torque limited/2(SpdGov_trqSet)
  CoPT_trqDesCompEng/1 -> inner torque limited/3(CoPT_trqDesCompEng)
  inner torque limited/1(CoETS_trqUnFltLtdSet) -> CoETS_trqUnFltLtdSet/1
  inner torque limited/2(trqinrLtdSet) -> trqinrLtdSet/1
  CoETS_TrqCalc_Inl2/1(CoETS_trqInrLim) -> inner torque limited/1(CoETS_trqInrLim), CoETS_trqInrLim/1

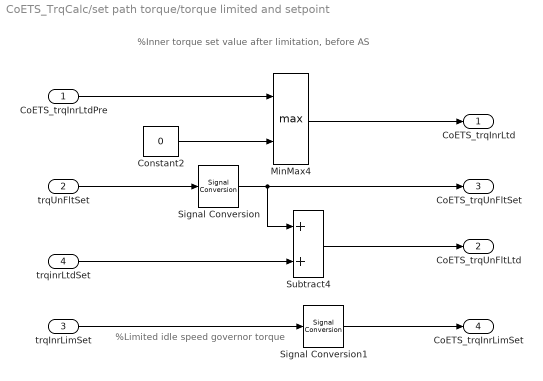
== system CoETS_TrqCalc/set path torque/torque limited and setpoint ==
  note: %Inner torque set value after limitation, before AS
  note: %Limited idle speed governor torque
  CoETS_trqInrLtdPre : Inport
  trqUnFltSet : Inport  Port=2
  trqInrLimSet : Inport  Port=3
  trqinrLtdSet : Inport  Port=4
  Constant2 : Constant  Value=0  VectorParams1D=off  OutDataTypeStr=Inherit: Inherit via back propagation
  MinMax4 : MinMax  Function=max  Inputs=2  InputSameDT=on
  Signal Conversion : SignalConversion  OverrideOpt=off
  Signal Conversion1 : SignalConversion  OverrideOpt=off
  Subtract4 : Sum  OutDataTypeStr=Inherit: Inherit via back propagation  SaturateOnIntegerOverflow=on  InputSameDT=on
  CoETS_trqInrLtd : Outport
  CoETS_trqUnFltLtd : Outport  Port=2
  CoETS_trqUnFltSet : Outport  Port=3
  CoETS_trqInrLimSet : Outport  Port=4
  wires:
  CoETS_trqInrLtdPre/1 -> MinMax4/1
  MinMax4/1 -> CoETS_trqInrLtd/1
  trqUnFltSet/1 -> Signal Conversion/1
  Constant2/1 -> MinMax4/2
  trqInrLimSet/1 -> Signal Conversion1/1
  Subtract4/1 -> CoETS_trqUnFltLtd/1
  trqinrLtdSet/1 -> Subtract4/2
  Signal Conversion/1 -> Subtract4/1, CoETS_trqUnFltSet/1
  Signal Conversion1/1 -> CoETS_trqInrLimSet/1

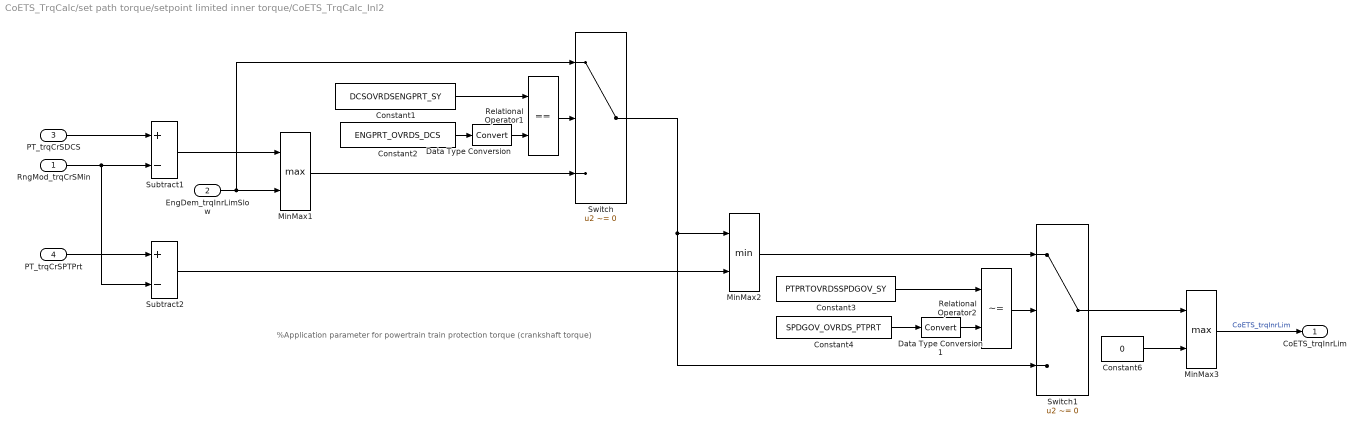
== system CoETS_TrqCalc/set path torque/setpoint limited inner torque/CoETS_TrqCalc_Inl2 ==
  note: %Application parameter for powertrain train protection torque (crankshaft torque)
  RngMod_trqCrSMin : Inport
  EngDem_trqInrLimSlow : Inport  Port=2
  PT_trqCrSDCS : Inport  Port=3
  PT_trqCrSPTPrt : Inport  Port=4
  Constant1 : Constant  Value=DCSOVRDSENGPRT_SY  VectorParams1D=off
  Constant2 : Constant  Value=ENGPRT_OVRDS_DCS  VectorParams1D=off
  Constant3 : Constant  Value=PTPRTOVRDSSPDGOV_SY  VectorParams1D=off
  Constant4 : Constant  Value=SPDGOV_OVRDS_PTPRT  VectorParams1D=off
  Constant6 : Constant  Value=0  VectorParams1D=off  OutDataTypeStr=Inherit: Inherit via back propagation
  Data Type Conversion : DataTypeConversion
  Data Type Conversion1 : DataTypeConversion
  MinMax1 : MinMax  Function=max  Inputs=2  InputSameDT=on
  MinMax2 : MinMax  Inputs=2  InputSameDT=on
  MinMax3 : MinMax  Function=max  Inputs=2  InputSameDT=on
  Relational Operator1 : RelationalOperator  Operator===  OutDataTypeStr=boolean  RndMeth=Simplest  InputSameDT=on
  Relational Operator2 : RelationalOperator  Operator=~=  OutDataTypeStr=boolean  RndMeth=Simplest  InputSameDT=on
  Subtract1 : Sum  Inputs=+-  OutDataTypeStr=Inherit: Inherit via back propagation  SaturateOnIntegerOverflow=on  InputSameDT=on
  Subtract2 : Sum  Inputs=+-  OutDataTypeStr=Inherit: Inherit via back propagation  SaturateOnIntegerOverflow=on  InputSameDT=on
  Switch : Switch  Criteria=u2 ~= 0  OutDataTypeStr=Inherit: Inherit via back propagation  SaturateOnIntegerOverflow=on  InputSameDT=on
  Switch1 : Switch  Criteria=u2 ~= 0  OutDataTypeStr=Inherit: Inherit via back propagation  SaturateOnIntegerOverflow=on  InputSameDT=on
  CoETS_trqInrLim : Outport
  wires:
  Data Type Conversion1/1 -> Relational Operator2/2
  Data Type Conversion/1 -> Relational Operator1/2
  MinMax3/1 -> CoETS_trqInrLim/1  "CoETS_trqInrLim"
  Constant6/1 -> MinMax3/2
  Switch1/1 -> MinMax3/1
  Relational Operator2/1 -> Switch1/2
  MinMax2/1 -> Switch1/1
  Switch/1 -> Switch1/3, MinMax2/1
  Subtract2/1 -> MinMax2/2
  RngMod_trqCrSMin/1 -> Subtract1/2, Subtract2/2
  PT_trqCrSPTPrt/1 -> Subtract2/1
  Relational Operator1/1 -> Switch/2
  MinMax1/1 -> Switch/3
  EngDem_trqInrLimSlow/1 -> MinMax1/2, Switch/1
  Subtract1/1 -> MinMax1/1
  PT_trqCrSDCS/1 -> Subtract1/1
  Constant4/1 -> Data Type Conversion1/1
  Constant3/1 -> Relational Operator2/1
  Constant2/1 -> Data Type Conversion/1
  Constant1/1 -> Relational Operator1/1

== system CoETS_TrqCalc/set path torque/setpoint limited inner torque/inner torque limited ==
  note: %Compensation torque of the accessories
  CoETS_trqInrLim : Inport
  SpdGov_trqSet : Inport  Port=2
  CoPT_trqDesCompEng : Inport  Port=3
  Constant1 : Constant  Value=0  VectorParams1D=off  OutDataTypeStr=Inherit: Inherit via back propagation
  MinMax1 : MinMax  Function=max  Inputs=2  InputSameDT=on
  MinMax2 : MinMax  Inputs=2  InputSameDT=on
  MinMax3 : MinMax  Inputs=2  InputSameDT=on
  Subtract1 : Sum  OutDataTypeStr=Inherit: Inherit via back propagation  SaturateOnIntegerOverflow=on  InputSameDT=on
  Subtract3 : Sum  OutDataTypeStr=Inherit: Inherit via back propagation  SaturateOnIntegerOverflow=on  InputSameDT=on
  CoETS_trqUnFltLtdSet : Outport
  trqinrLtdSet : Outport  Port=2
  wires:
  MinMax1/1 -> Subtract1/1
  MinMax3/1 -> trqinrLtdSet/1
  Subtract3/1 -> MinMax3/2
  Subtract1/1 -> MinMax2/2
  CoPT_trqDesCompEng/1 -> Subtract1/2, Subtract3/1
  Constant1/1 -> MinMax1/2
  SpdGov_trqSet/1 -> MinMax1/1, Subtract3/2
  MinMax2/1 -> CoETS_trqUnFltLtdSet/1
  CoETS_trqInrLim/1 -> MinMax3/1, MinMax2/1
